simulink model "SGP_to_GPS"  (R2015b)
settings: Solver=VariableStepAuto  StartTime=0.0  StopTime=20000  RelTol=1e-3
undefined symbols (not defined in the file): Earth, equinox, s_SIM_STEP_SIZE, TLE_epoch, today, Ts_display, WGS84
libraries: xpcutilitieslib x17, aerolibtransform2 x1
settings Model: Creator=Rohit Engl  LastModifiedBy=Rohit Engl

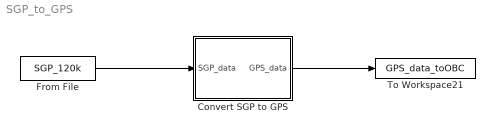
== system SGP_to_GPS ==
  Convert SGP to GPS : Subsystem
  From File : FromFile  FileName=SGP_120k  SampleTime=s_SIM_STEP_SIZE
  To Workspace21 : ToWorkspace  VariableName=GPS_data_toOBC  SampleTime=-1
      settings: MaxDataPoints=1
  wires:
  From File/1 -> Convert SGP to GPS/1(SGP_data)
  Convert SGP to GPS/1(GPS_data) -> To Workspace21/1

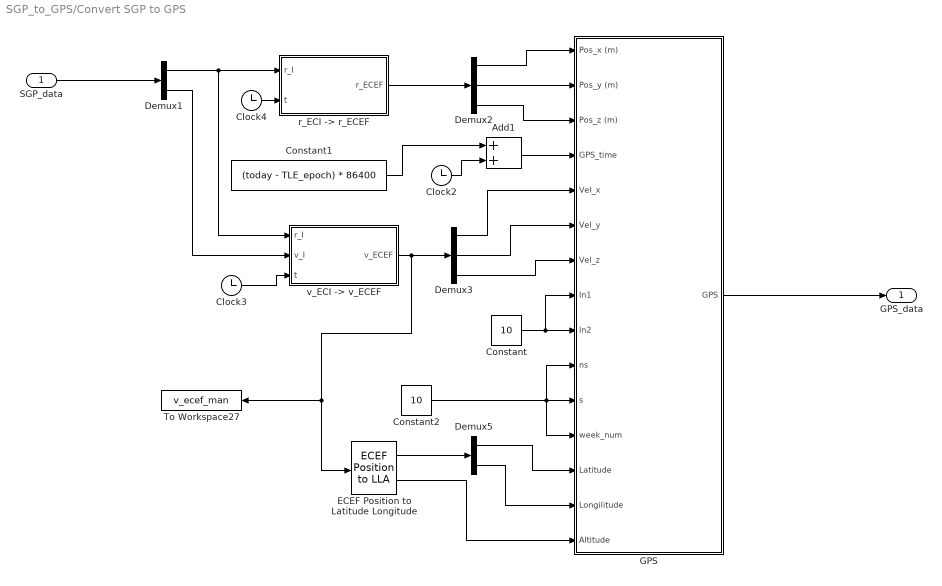
== system SGP_to_GPS/Convert SGP to GPS ==
  SGP_data : Inport
  Add1 : Sum
  Clock2 : Clock
  Clock3 : Clock
  Clock4 : Clock
  Constant : Constant  Value=10  OutDataTypeStr=uint8
  Constant1 : Constant  Value=(today - TLE_epoch) * 86400  VectorParams1D=off
  Constant2 : Constant  Value=10  OutDataTypeStr=double
  Demux1 : Demux  Outputs=2
  Demux2 : Demux  Outputs=3
  Demux3 : Demux  Outputs=3
  Demux5 : Demux  Outputs=2
  ECEF Position to Latitude Longitude : aerolibtransform2/ECEF Position to LLA  units=Metric (MKS)  ptype=Earth (WGS84)  F=1/298.257223563  R=6378137
  GPS : Subsystem
  To Workspace27 : ToWorkspace  VariableName=v_ecef_man  SampleTime=Ts_display
  "r_ECI -> r_ECEF" : MATLAB Function  TreatAsAtomicUnit=on
  "v_ECI -> v_ECEF" : MATLAB Function  TreatAsAtomicUnit=on
  GPS_data : Outport
  wires:
  Constant/1 -> GPS/9(In2), GPS/8(In1)
  ECEF Position to Latitude Longitude/1 -> Demux5/1
  ECEF Position to Latitude Longitude/2 -> GPS/15(Altitude)
  Constant2/1 -> GPS/10(ns), GPS/12(week_num), GPS/11(s)
  Demux5/1 -> GPS/13(Latitude)
  GPS/1(GPS) -> GPS_data/1
  Demux5/2 -> GPS/14("Longilitude ")
  Constant1/1 -> Add1/1
  Clock2/1 -> Add1/2
  Add1/1 -> GPS/4(GPS_time)
  Demux1/2 -> "v_ECI -> v_ECEF"/2(v_I)
  "v_ECI -> v_ECEF"/1(v_ECEF) -> Demux3/1, ECEF Position to Latitude Longitude/1, To Workspace27/1
  Demux3/1 -> GPS/5(Vel_x)
  Demux3/2 -> GPS/6(Vel_y)
  Clock3/1 -> "v_ECI -> v_ECEF"/3(t)
  Demux3/3 -> GPS/7(Vel_z)
  "r_ECI -> r_ECEF"/1(r_ECEF) -> Demux2/1
  Demux2/1 -> GPS/1(Pos_x (m))
  Demux2/2 -> GPS/2(Pos_y (m))
  Demux2/3 -> GPS/3(Pos_z (m))
  Demux1/1 -> "v_ECI -> v_ECEF"/1(r_I), "r_ECI -> r_ECEF"/1(r_I)
  SGP_data/1 -> Demux1/1
  Clock4/1 -> "r_ECI -> r_ECEF"/2(t)

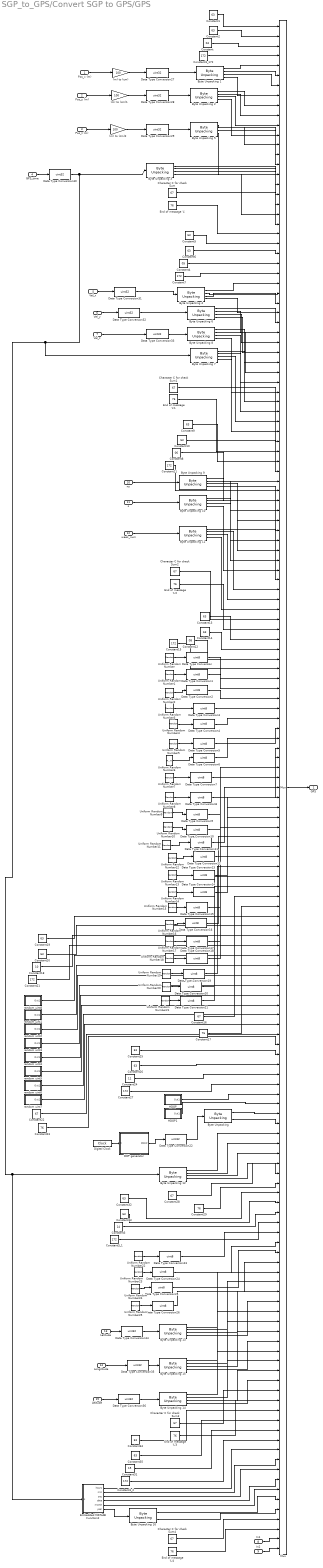
== system SGP_to_GPS/Convert SGP to GPS/GPS ==
  Pos_x (m) : Inport
  Pos_y (m) : Inport  Port=2
  Pos_z (m) : Inport  Port=3
  GPS_time : Inport  Port=4
  Vel_x : Inport  Port=5
  Vel_y : Inport  Port=6
  Vel_z : Inport  Port=7
  In1 : Inport  Port=8  OutDataTypeStr=uint8
  In2 : Inport  Port=9  OutDataTypeStr=uint8
  ns : Inport  Port=10
  s : Inport  Port=11
  week_num : Inport  Port=12
  Latitude : Inport  Port=13
  "Longilitude " : Inport  Port=14
  Altitude : Inport  Port=15
  (m) to (cm) : Gain  Gain=100  OutDataTypeStr=double
  (m) to (cm)1 : Gain  Gain=100
  (m) to (cm)2 : Gain  Gain=100
  Byte Unpacking {,1..16} (17 alike) : xpcutilitieslib/Byte Unpacking 
  Character C for check Sum{,1..4} (5 alike) : Constant  Value=67  OutDataTypeStr=uint8
  Constant : Constant  Value=04  OutDataTypeStr=uint8
  Constant{1..2,5..6,9..10,13..14,19..20,25..26,32..35} (16 alike) : Constant  Value=63  OutDataTypeStr=uint8
  Constant{7,11,15,21,27} (5 alike) : Constant  Value=172  OutDataTypeStr=uint8
  Constant12 : Constant  Value=08  OutDataTypeStr=uint8
  Constant16 : Constant  Value=67  OutDataTypeStr=uint8
  Constant17 : Constant  Value=76  OutDataTypeStr=uint8
  Constant18 : Constant  Value=10  OutDataTypeStr=uint8
  Constant22 : Constant  Value=67  OutDataTypeStr=uint8
  Constant23 : Constant  Value=76  OutDataTypeStr=uint8
  Constant24 : Constant  Value=11  OutDataTypeStr=uint8
  Constant28 : Constant  Value=67  OutDataTypeStr=uint8
  Constant29 : Constant  Value=76  OutDataTypeStr=uint8
  Constant3 : Constant  Value=14  OutDataTypeStr=uint8
  Constant31 : Constant  Value=15  OutDataTypeStr=uint8
  Constant3_1 : Constant  Value=172  OutDataTypeStr=uint8
  Constant3_172 : Constant  Value=172  OutDataTypeStr=uint8
  Constant3_2 : Constant  Value=172  OutDataTypeStr=uint8
  Constant4 : Constant  Value=05  OutDataTypeStr=uint8
  Constant8 : Constant  Value=06  OutDataTypeStr=uint8
  DOP generator : MATLAB Function  TreatAsAtomicUnit=on
  Data Type Conversion{,1..21,23..26} (26 alike) : DataTypeConversion  OutDataTypeStr=uint8
  Data Type Conversion{22,27..36} (11 alike) : DataTypeConversion  OutDataTypeStr=uint32
  Digital Clock : DigitalClock  SampleTime=0.1
  Embedded MATLAB Function2 : MATLAB Function  TreatAsAtomicUnit=on
  End of message 'L'{,1..4} (5 alike) : Constant  Value=76  OutDataTypeStr=uint8
  HDOP : Subsystem
  HDOP1 : Subsystem
  Mux : Mux  Inputs=155
  Uniform Random Number{,1..25} (26 alike) : UniformRandomNumber  Minimum=0  Maximum=256  Seed=1  SampleTime=0.1
  random uint1 : Subsystem
  random uint2 : Subsystem
  random uint3 : Subsystem
  random uint4 : Subsystem
  random uint5 : Subsystem
  random uint6 : Subsystem
  random uint7 : Subsystem
  random uint8 : Subsystem
  GPS : Outport
  wires:
  Constant1/1 -> Mux/1
  Constant2/1 -> Mux/2
  Constant/1 -> Mux/3
  Constant3_172/1 -> Mux/4
  GPS_time/1 -> Data Type Conversion30/1
  Byte Unpacking 3/1 -> Mux/17
  Byte Unpacking 3/2 -> Mux/18
  Byte Unpacking 3/3 -> Mux/19
  Character C for check Sum/1 -> Mux/21
  End of message 'L'/1 -> Mux/22
  Byte Unpacking 3/4 -> Mux/20
  Pos_x (m)/1 -> (m) to (cm)/1
  Pos_y (m)/1 -> (m) to (cm)1/1
  Pos_z (m)/1 -> (m) to (cm)2/1
  Byte Unpacking 5/1 -> Mux/13
  Byte Unpacking 5/2 -> Mux/14
  Byte Unpacking 5/3 -> Mux/15
  Byte Unpacking 5/4 -> Mux/16
  Byte Unpacking 1/1 -> Mux/5
  Byte Unpacking 1/2 -> Mux/6
  Byte Unpacking 1/3 -> Mux/7
  Byte Unpacking 1/4 -> Mux/8
  Byte Unpacking 2/1 -> Mux/9
  Byte Unpacking 2/2 -> Mux/10
  Byte Unpacking 2/3 -> Mux/11
  Byte Unpacking 2/4 -> Mux/12
  Constant5/1 -> Mux/23
  Constant6/1 -> Mux/24
  Constant4/1 -> Mux/25
  Constant7/1 -> Mux/26
  Byte Unpacking 4/1 -> Mux/27
  Byte Unpacking 4/2 -> Mux/28
  Byte Unpacking 4/3 -> Mux/29
  Byte Unpacking 4/4 -> Mux/30
  Byte Unpacking 6/1 -> Mux/31
  Byte Unpacking 6/2 -> Mux/32
  Byte Unpacking 6/3 -> Mux/33
  Byte Unpacking 6/4 -> Mux/34
  Byte Unpacking 8/1 -> Mux/35
  Byte Unpacking 8/2 -> Mux/36
  Byte Unpacking 8/3 -> Mux/37
  Byte Unpacking 8/4 -> Mux/38
  Byte Unpacking 7/1 -> Mux/39
  Byte Unpacking 7/2 -> Mux/40
  Byte Unpacking 7/3 -> Mux/41
  Byte Unpacking 7/4 -> Mux/42
  Character C for check Sum1/1 -> Mux/43
  End of message 'L'1/1 -> Mux/44
  Constant9/1 -> Mux/45
  Constant10/1 -> Mux/46
  Constant8/1 -> Mux/47
  Constant11/1 -> Mux/48
  Byte Unpacking 9/1 -> Mux/49
  Byte Unpacking 9/2 -> Mux/50
  Byte Unpacking 9/3 -> Mux/51
  Byte Unpacking 9/4 -> Mux/52
  Byte Unpacking 10/1 -> Mux/53
  Byte Unpacking 10/2 -> Mux/54
  Byte Unpacking 10/3 -> Mux/55
  Byte Unpacking 10/4 -> Mux/56
  Byte Unpacking 11/1 -> Mux/57
  Byte Unpacking 11/2 -> Mux/58
  Byte Unpacking 11/3 -> Mux/59
  Byte Unpacking 11/4 -> Mux/60
  Character C for check Sum2/1 -> Mux/61
  End of message 'L'2/1 -> Mux/62
  Uniform Random Number/1 -> Data Type Conversion/1
  Uniform Random Number1/1 -> Data Type Conversion1/1
  Uniform Random Number2/1 -> Data Type Conversion2/1
  Uniform Random Number3/1 -> Data Type Conversion3/1
  Uniform Random Number4/1 -> Data Type Conversion4/1
  Uniform Random Number5/1 -> Data Type Conversion5/1
  Uniform Random Number6/1 -> Data Type Conversion6/1
  Uniform Random Number7/1 -> Data Type Conversion7/1
  Uniform Random Number8/1 -> Data Type Conversion8/1
  Uniform Random Number9/1 -> Data Type Conversion9/1
  Uniform Random Number10/1 -> Data Type Conversion10/1
  Uniform Random Number11/1 -> Data Type Conversion11/1
  Uniform Random Number12/1 -> Data Type Conversion12/1
  Uniform Random Number13/1 -> Data Type Conversion13/1
  Uniform Random Number14/1 -> Data Type Conversion14/1
  Uniform Random Number15/1 -> Data Type Conversion15/1
  Uniform Random Number16/1 -> Data Type Conversion16/1
  Uniform Random Number17/1 -> Data Type Conversion17/1
  Uniform Random Number18/1 -> Data Type Conversion18/1
  Uniform Random Number19/1 -> Data Type Conversion19/1
  Uniform Random Number20/1 -> Data Type Conversion20/1
  Uniform Random Number21/1 -> Data Type Conversion21/1
  Constant13/1 -> Mux/63
  Constant14/1 -> Mux/64
  Constant12/1 -> Mux/65
  Constant15/1 -> Mux/66
  Data Type Conversion/1 -> Mux/67
  Data Type Conversion1/1 -> Mux/68
  Data Type Conversion2/1 -> Mux/69
  Data Type Conversion3/1 -> Mux/70
  Data Type Conversion4/1 -> Mux/71
  Data Type Conversion5/1 -> Mux/72
  Data Type Conversion6/1 -> Mux/73
  Data Type Conversion7/1 -> Mux/74
  Data Type Conversion8/1 -> Mux/75
  Data Type Conversion9/1 -> Mux/76
  Data Type Conversion10/1 -> Mux/77
  Data Type Conversion11/1 -> Mux/78
  Data Type Conversion12/1 -> Mux/79
  Data Type Conversion13/1 -> Mux/80
  Data Type Conversion14/1 -> Mux/81
  Data Type Conversion15/1 -> Mux/82
  Data Type Conversion16/1 -> Mux/83
  Data Type Conversion17/1 -> Mux/84
  Data Type Conversion18/1 -> Mux/85
  Data Type Conversion19/1 -> Mux/86
  Data Type Conversion20/1 -> Mux/87
  Data Type Conversion21/1 -> Mux/88
  Constant16/1 -> Mux/89
  Constant17/1 -> Mux/90
  Digital Clock/1 -> DOP generator/1(t)
  DOP generator/1(PDOP) -> Data Type Conversion22/1
  Data Type Conversion22/1 -> "Byte Unpacking "/1
  ns/1 -> Byte Unpacking 9/1
  s/1 -> Byte Unpacking 10/1
  week_num/1 -> Byte Unpacking 11/1
  Uniform Random Number22/1 -> Data Type Conversion23/1
  Uniform Random Number23/1 -> Data Type Conversion24/1
  Uniform Random Number24/1 -> Data Type Conversion25/1
  Uniform Random Number25/1 -> Data Type Conversion26/1
  Constant19/1 -> Mux/91
  Constant20/1 -> Mux/92
  Constant18/1 -> Mux/93
  Constant21/1 -> Mux/94
  random uint8/1(Out1) -> Mux/95
  random uint1/1(Out1) -> Mux/96
  random uint2/1(Out1) -> Mux/97
  random uint3/1(Out1) -> Mux/98
  random uint4/1(Out1) -> Mux/99
  random uint5/1(Out1) -> Mux/100
  random uint6/1(Out1) -> Mux/101
  random uint7/1(Out1) -> Mux/102
  Constant22/1 -> Mux/103
  Constant23/1 -> Mux/104
  Constant25/1 -> Mux/105
  Constant26/1 -> Mux/106
  Constant24/1 -> Mux/107
  Constant27/1 -> Mux/108
  HDOP/1(Out1) -> Mux/109
  HDOP1/1(Out1) -> Mux/110
  "Byte Unpacking "/1 -> Mux/111
  "Byte Unpacking "/2 -> Mux/112
  Byte Unpacking 12/1 -> Mux/113
  Byte Unpacking 12/2 -> Mux/114
  Byte Unpacking 12/3 -> Mux/115
  Byte Unpacking 12/4 -> Mux/116
  Constant28/1 -> Mux/117
  Constant29/1 -> Mux/118
  Constant32/1 -> Mux/119
  Constant33/1 -> Mux/120
  Constant3/1 -> Mux/121
  Constant3_1/1 -> Mux/122
  Data Type Conversion23/1 -> Mux/123
  Data Type Conversion24/1 -> Mux/124
  Data Type Conversion25/1 -> Mux/125
  Data Type Conversion26/1 -> Mux/126
  Byte Unpacking 13/1 -> Mux/127
  Byte Unpacking 13/2 -> Mux/128
  Byte Unpacking 13/3 -> Mux/129
  Byte Unpacking 13/4 -> Mux/130
  Byte Unpacking 15/1 -> Mux/131
  Byte Unpacking 15/2 -> Mux/132
  Byte Unpacking 15/3 -> Mux/133
  Byte Unpacking 15/4 -> Mux/134
  Byte Unpacking 14/1 -> Mux/135
  Byte Unpacking 14/2 -> Mux/136
  Byte Unpacking 14/3 -> Mux/137
  Byte Unpacking 14/4 -> Mux/138
  Character C for check Sum3/1 -> Mux/139
  End of message 'L'3/1 -> Mux/140
  Constant34/1 -> Mux/141
  Constant35/1 -> Mux/142
  Constant31/1 -> Mux/143
  Constant3_2/1 -> Mux/144
  Embedded MATLAB Function2/1(hours) -> Mux/145
  Embedded MATLAB Function2/2(min) -> Mux/146
  Embedded MATLAB Function2/3(sec) -> Mux/147
  Embedded MATLAB Function2/4(date) -> Mux/148
  Embedded MATLAB Function2/5(month) -> Mux/149
  In1/1 -> Mux/154
  In2/1 -> Mux/155
  End of message 'L'4/1 -> Mux/153
  Character C for check Sum4/1 -> Mux/152
  Embedded MATLAB Function2/6(year) -> Byte Unpacking 16/1
  Byte Unpacking 16/1 -> Mux/150
  Byte Unpacking 16/2 -> Mux/151
  Data Type Conversion27/1 -> Byte Unpacking 1/1
  Data Type Conversion28/1 -> Byte Unpacking 2/1
  Data Type Conversion29/1 -> Byte Unpacking 5/1
  Data Type Conversion30/1 -> Byte Unpacking 3/1, Byte Unpacking 7/1, Byte Unpacking 12/1, Embedded MATLAB Function2/1(s)
  (m) to (cm)/1 -> Data Type Conversion27/1
  (m) to (cm)1/1 -> Data Type Conversion28/1
  (m) to (cm)2/1 -> Data Type Conversion29/1
  Vel_z/1 -> Data Type Conversion33/1
  Data Type Conversion33/1 -> Byte Unpacking 8/1
  Vel_y/1 -> Data Type Conversion32/1
  Data Type Conversion32/1 -> Byte Unpacking 6/1
  Vel_x/1 -> Data Type Conversion31/1
  Data Type Conversion31/1 -> Byte Unpacking 4/1
  Latitude/1 -> Data Type Conversion34/1
  Data Type Conversion34/1 -> Byte Unpacking 13/1
  Altitude/1 -> Data Type Conversion36/1
  Data Type Conversion36/1 -> Byte Unpacking 14/1
  "Longilitude "/1 -> Data Type Conversion35/1
  Data Type Conversion35/1 -> Byte Unpacking 15/1
  Mux/1 -> GPS/1

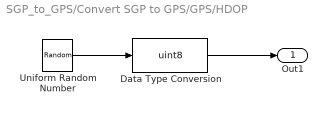
== system SGP_to_GPS/Convert SGP to GPS/GPS/HDOP ==
  Data Type Conversion : DataTypeConversion  OutDataTypeStr=uint8
  Uniform Random Number : UniformRandomNumber  Minimum=0  Maximum=256  SampleTime=0.1
  Out1 : Outport
  wires:
  Uniform Random Number/1 -> Data Type Conversion/1
  Data Type Conversion/1 -> Out1/1

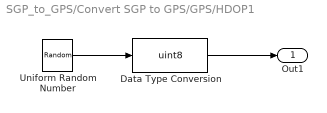
== system SGP_to_GPS/Convert SGP to GPS/GPS/HDOP1 ==
  Data Type Conversion : DataTypeConversion  OutDataTypeStr=uint8
  Uniform Random Number : UniformRandomNumber  Minimum=0  Maximum=256  SampleTime=0.1
  Out1 : Outport
  wires:
  Uniform Random Number/1 -> Data Type Conversion/1
  Data Type Conversion/1 -> Out1/1

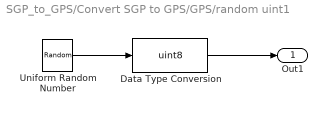
== system SGP_to_GPS/Convert SGP to GPS/GPS/random uint1 ==
  Data Type Conversion : DataTypeConversion  OutDataTypeStr=uint8
  Uniform Random Number : UniformRandomNumber  Minimum=0  Maximum=256  SampleTime=0.1
  Out1 : Outport
  wires:
  Uniform Random Number/1 -> Data Type Conversion/1
  Data Type Conversion/1 -> Out1/1

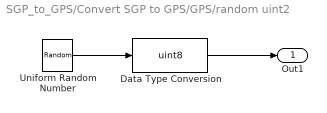
== system SGP_to_GPS/Convert SGP to GPS/GPS/random uint2 ==
  Data Type Conversion : DataTypeConversion  OutDataTypeStr=uint8
  Uniform Random Number : UniformRandomNumber  Minimum=0  Maximum=256  SampleTime=0.1
  Out1 : Outport
  wires:
  Uniform Random Number/1 -> Data Type Conversion/1
  Data Type Conversion/1 -> Out1/1

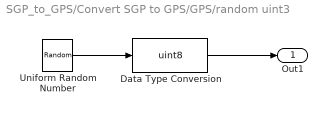
== system SGP_to_GPS/Convert SGP to GPS/GPS/random uint3 ==
  Data Type Conversion : DataTypeConversion  OutDataTypeStr=uint8
  Uniform Random Number : UniformRandomNumber  Minimum=0  Maximum=256  SampleTime=0.1
  Out1 : Outport
  wires:
  Uniform Random Number/1 -> Data Type Conversion/1
  Data Type Conversion/1 -> Out1/1

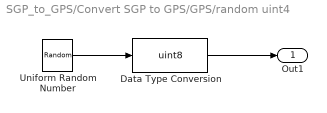
== system SGP_to_GPS/Convert SGP to GPS/GPS/random uint4 ==
  Data Type Conversion : DataTypeConversion  OutDataTypeStr=uint8
  Uniform Random Number : UniformRandomNumber  Minimum=0  Maximum=256  SampleTime=0.1
  Out1 : Outport
  wires:
  Uniform Random Number/1 -> Data Type Conversion/1
  Data Type Conversion/1 -> Out1/1

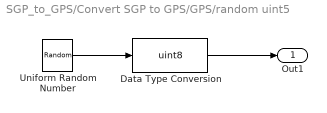
== system SGP_to_GPS/Convert SGP to GPS/GPS/random uint5 ==
  Data Type Conversion : DataTypeConversion  OutDataTypeStr=uint8
  Uniform Random Number : UniformRandomNumber  Minimum=0  Maximum=256  SampleTime=0.1
  Out1 : Outport
  wires:
  Uniform Random Number/1 -> Data Type Conversion/1
  Data Type Conversion/1 -> Out1/1

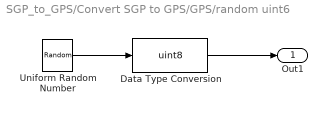
== system SGP_to_GPS/Convert SGP to GPS/GPS/random uint6 ==
  Data Type Conversion : DataTypeConversion  OutDataTypeStr=uint8
  Uniform Random Number : UniformRandomNumber  Minimum=0  Maximum=256  SampleTime=0.1
  Out1 : Outport
  wires:
  Uniform Random Number/1 -> Data Type Conversion/1
  Data Type Conversion/1 -> Out1/1

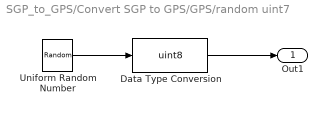
== system SGP_to_GPS/Convert SGP to GPS/GPS/random uint7 ==
  Data Type Conversion : DataTypeConversion  OutDataTypeStr=uint8
  Uniform Random Number : UniformRandomNumber  Minimum=0  Maximum=256  SampleTime=0.1
  Out1 : Outport
  wires:
  Uniform Random Number/1 -> Data Type Conversion/1
  Data Type Conversion/1 -> Out1/1

== system SGP_to_GPS/Convert SGP to GPS/GPS/random uint8 ==
  Data Type Conversion : DataTypeConversion  OutDataTypeStr=uint8
  Uniform Random Number : UniformRandomNumber  Minimum=0  Maximum=256  SampleTime=0.1
  Out1 : Outport
  wires:
  Uniform Random Number/1 -> Data Type Conversion/1
  Data Type Conversion/1 -> Out1/1

== matlab function SGP_to_GPS/Convert SGP to GPS/GPS/DOP generator ==
  data: t input; PDOP output
function PDOP = gen_dop(t)
%#eml\

if (t < 70)
    DOP = 100 - (1.4*(t));
    random = 10*randn();
    PDOP = DOP + random;
else
    DOP = 1;
    random = 0.5*(randn());
    PDOP = DOP + random;
end

== matlab function SGP_to_GPS/Convert SGP to GPS/GPS/Embedded MATLAB Function2 ==
  data: hours output; min output; sec output; date output; month output; s input; year output
function [hours,min,sec,date,month,year] = fcn(s)

%#eml
%temp = datevec(date);

hours = uint8(rem(s/3600,24)+10);
min = uint8(rem(s/60,60)+30);
sec = uint8(rem(s,60));


date = uint8(18); %uint8(temp(3));
month = uint8(10); % uint8(temp(2));
year = uint16(2015); %uint16(temp(1));

== matlab function SGP_to_GPS/Convert SGP to GPS/r_ECI -> r_ECEF ==
  data: today parameter; r_ECEF output; equinox parameter; r_I input; t input
function r_ECEF = fcn(today,equinox,r_I,t)
%u: position vector in ECI (in m)
%y: position vector in ECEF (in m)

stperut = 1.00273790935;    % siderial time = stperut * universal time
W_EARTH_ROT = 2*pi/86141;   % sidereal rotation angular velocity of earth, SI

ut_sec = (today - equinox)*24*60*60 + t; % universal time vector in sec
st_sec = stperut*ut_sec;    % sidereal time vector in sec

phi = st_sec*W_EARTH_ROT;            % sidereal time vector in rad

TEI = [ cos(phi) sin(phi) 0;
       -sin(phi) cos(phi) 0;
        0        0        1];

r_ECEF = TEI*r_I;

== matlab function SGP_to_GPS/Convert SGP to GPS/v_ECI -> v_ECEF ==
  data: today parameter; v_ECEF output; equinox parameter; r_I input; v_I input; t input
function v_ECEF = fcn(today,equinox,r_I,v_I,t)
%u: position vector in ECI (in m)
%y: position vector in ECEF (in m)

stperut = 1.00273790935;    % siderial time = stperut * universal time
W_EARTH_ROT = 2*pi/86141;   % sidereal rotation angular velocity of earth, SI

ut_sec = (today - equinox)*24*60*60 + t; % universal time vector in sec
st_sec = stperut*ut_sec;    % sidereal time vector in sec

phi = st_sec*W_EARTH_ROT;            % sidereal time vector in rad

TEI = [ cos(phi) sin(phi) 0;
       -sin(phi) cos(phi) 0;
        0        0        1];

phi_dot = W_EARTH_ROT;    

TEI_dot = phi_dot* [ -sin(phi)  cos(phi) 0;
                     -cos(phi) -sin(phi) 0;
                      0         0        0];
    
    
v_ECEF = TEI*v_I + TEI_dot*r_I;
